simulink model "AM"  (R2016a)
settings: Solver=ode3  StartTime=0.0  StopTime=0.025  FixedStep=1/100000  RelTol=1e-3
libraries: dsparch4 x1
settings Model: Creator=camj3302  LastModifiedBy=camj3302
settings SolverCC: AutoInsertRateTranBlk=on

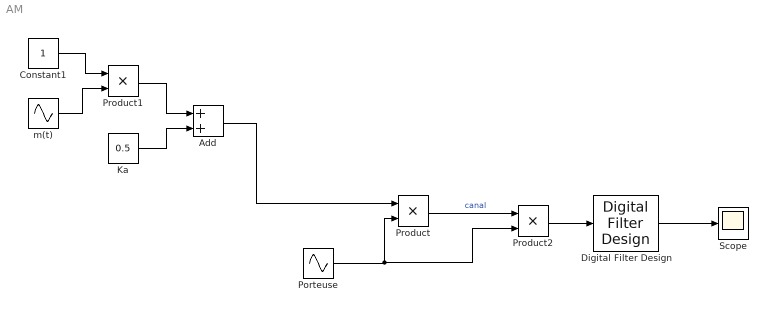
== system AM ==
  Add : Sum
  Constant1 : Constant  SampleTime=-1
  Digital Filter Design : dsparch4/Digital Filter Design  mwdsp_browser_bugfix_var=off
  Ka : Constant  Value=0.5  SampleTime=-1
  Porteuse : Sin  Frequency=10000*2*pi  Phase=pi/2  SampleTime=0
  Product : Product
  Product1 : Product
  Product2 : Product
  Scope : Scope
  m(t) : Sin  Frequency=200*2*pi  SampleTime=0
  wires:
  Constant1/1 -> Product1/1
  m(t)/1 -> Product1/2
  Product1/1 -> Add/1
  Ka/1 -> Add/2
  Porteuse/1 -> Product/2, Product2/2
  Product/1 -> Product2/1  "canal"
  Product2/1 -> Digital Filter Design/1
  Add/1 -> Product/1
  Digital Filter Design/1 -> Scope/1
